simulink model "q1_b"  (R2026a)
settings: Solver=VariableStepAuto
model workspace (MAT data in the model file):
  K = Simulink.Parameter
  K.Complexity = 'real'
  K.Dimensions = [0 0]
  K.DataType = 'auto'
  K1 = Simulink.Parameter
  K1.Value = 4
  K1.Complexity = 'real'
  K1.Dimensions = [1 1]
  K1.DataType = 'auto'
  K1_2 = Simulink.Parameter
  K1_2.Value = 2
  K1_2.Complexity = 'real'
  K1_2.Dimensions = [1 1]
  K1_2.DataType = 'auto'
  K1_3 = Simulink.Parameter
  K1_3.Value = 5
  K1_3.Complexity = 'real'
  K1_3.Dimensions = [1 1]
  K1_3.DataType = 'auto'
  K2 = Simulink.Parameter
  K2.Value = 2
  K2.Complexity = 'real'
  K2.Dimensions = [1 1]
  K2.DataType = 'auto'
  K2_2 = Simulink.Parameter
  K2_2.Value = 4
  K2_2.Complexity = 'real'
  K2_2.Dimensions = [1 1]
  K2_2.DataType = 'auto'
  K2_3 = Simulink.Parameter
  K2_3.Value = 10
  K2_3.Complexity = 'real'
  K2_3.Dimensions = [1 1]
  K2_3.DataType = 'auto'
  a = Simulink.Parameter
  a.Value = 2
  a.Complexity = 'real'
  a.Dimensions = [1 1]
  a.DataType = 'auto'
settings Model: Creator=LAB_PC  LastModifiedBy=LAB_PC

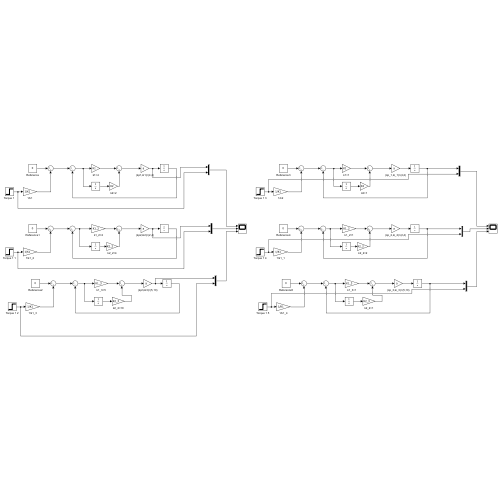
[thumbnail: Simulink's stored preview of the top-level diagram]
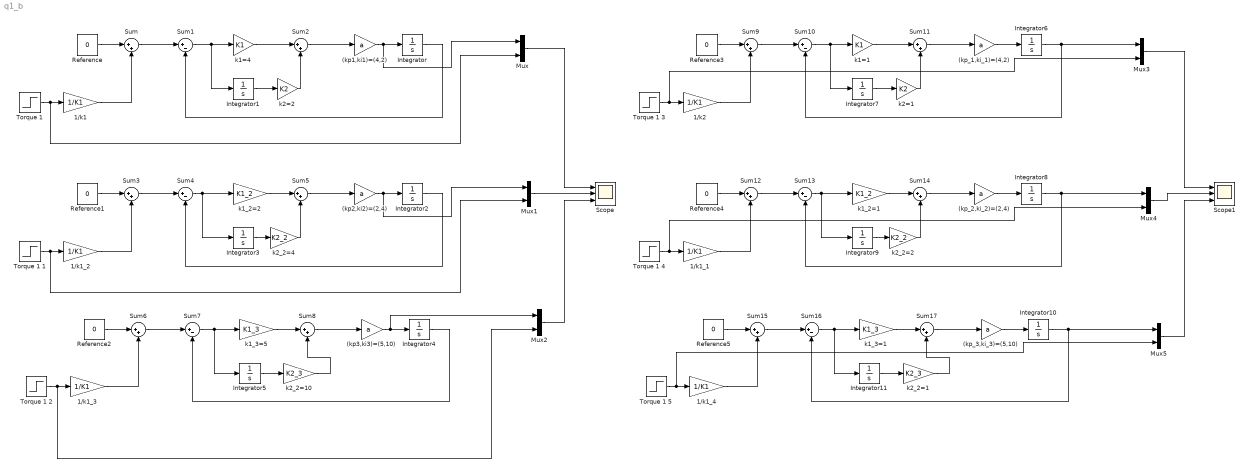
== system q1_b ==
  (kp1,ki1)=(4,2) : Gain  Gain=a
  (kp2,ki2)=(2,4) : Gain  Gain=a
  (kp3,ki3)=(5,10) : Gain  Gain=a
  (kp_1,ki_1)=(4,2) : Gain  Gain=a
  (kp_2,ki_2)=(2,4) : Gain  Gain=a
  (kp_3,ki_3)=(5,10) : Gain  Gain=a
  1/k1 : Gain  Gain=1/K1
  1/k1_{1..4} (4 alike) : Gain  Gain=1/K1
  1/k2 : Gain  Gain=1/K1
  Integrator{,1..11} (12 alike) : Integrator
  Mux{,1..5} (6 alike) : Mux  Inputs=2
  Reference{,1..5} (6 alike) : Constant  Value=0
  Scope : Scope  NumInputPorts=3
      settings: TimeAxisLabels=None  ActiveDisplayYMinimum=-3.7287146935324462  ActiveDisplayYMaximum=4.3917788582215262  DataLoggingVariableName=ScopeData2
  Scope1 : Scope  NumInputPorts=3
      settings: TimeAxisLabels=None  ActiveDisplayYMinimum=-3.7287146935324462  ActiveDisplayYMaximum=4.3917788582215262
  Sum{,2..3,5..6,8..9,11..12,14..15,17} (12 alike) : Sum  Inputs=|++
  Sum{1,4,7,10,13,16} (6 alike) : Sum  Inputs=|+-
  Torque 1 {,1..5} (6 alike) : Step  SampleTime=0
  k1=1 : Gain  Gain=K1
  k1=4 : Gain  Gain=K1
  k1_2=1 : Gain  Gain=K1_2
  k1_2=2 : Gain  Gain=K1_2
  k1_3=1 : Gain  Gain=K1_3
  k1_3=5 : Gain  Gain=K1_3
  k2=1 : Gain  Gain=K2
  k2=2 : Gain  Gain=K2
  k2_2=1 : Gain  Gain=K2_3
  k2_2=10 : Gain  Gain=K2_3
  k2_2=2 : Gain  Gain=K2_2
  k2_2=4 : Gain  Gain=K2_2
  wires:
  Integrator/1 -> Sum1/2
  Reference/1 -> Sum/1
  1/k1/1 -> Sum/2
  (kp1,ki1)=(4,2)/1 -> Mux/1, Integrator/1
  "Torque 1 "/1 -> Mux/2, 1/k1/1
  Mux/1 -> Scope/1
  Sum1/1 -> Integrator1/1, k1=4/1
  Sum/1 -> Sum1/1
  Integrator1/1 -> k2=2/1
  k2=2/1 -> Sum2/2
  k1=4/1 -> Sum2/1
  Sum2/1 -> (kp1,ki1)=(4,2)/1
  Integrator3/1 -> k2_2=4/1
  Sum3/1 -> Sum4/1
  Torque 1 1/1 -> Mux1/2, 1/k1_2/1
  k1_2=2/1 -> Sum5/1
  Sum5/1 -> (kp2,ki2)=(2,4)/1
  Integrator2/1 -> Sum4/2
  Reference1/1 -> Sum3/1
  Sum4/1 -> Integrator3/1, k1_2=2/1
  1/k1_2/1 -> Sum3/2
  k2_2=4/1 -> Sum5/2
  (kp2,ki2)=(2,4)/1 -> Mux1/1, Integrator2/1
  Sum6/1 -> Sum7/1
  (kp3,ki3)=(5,10)/1 -> Mux2/1, Integrator4/1
  k2_2=10/1 -> Sum8/2
  Sum7/1 -> Integrator5/1, k1_3=5/1
  1/k1_3/1 -> Sum6/2
  Integrator4/1 -> Sum7/2
  Reference2/1 -> Sum6/1
  Torque 1 2/1 -> Mux2/2, 1/k1_3/1
  Integrator5/1 -> k2_2=10/1
  k1_3=5/1 -> Sum8/1
  Sum8/1 -> (kp3,ki3)=(5,10)/1
  Mux1/1 -> Scope/2
  Mux2/1 -> Scope/3
  Mux4/1 -> Scope1/2
  Integrator6/1 -> Sum10/2, Mux3/1
  Sum14/1 -> (kp_2,ki_2)=(2,4)/1
  Integrator11/1 -> k2_2=1/1
  Sum11/1 -> (kp_1,ki_1)=(4,2)/1
  Torque 1 5/1 -> Mux5/2, 1/k1_4/1
  Mux5/1 -> Scope1/3
  (kp_3,ki_3)=(5,10)/1 -> Integrator10/1
  (kp_2,ki_2)=(2,4)/1 -> Integrator8/1
  Sum15/1 -> Sum16/1
  Sum12/1 -> Sum13/1
  Integrator7/1 -> k2=1/1
  Integrator8/1 -> Sum13/2, Mux4/1
  (kp_1,ki_1)=(4,2)/1 -> Integrator6/1
  Sum13/1 -> Integrator9/1, k1_2=1/1
  1/k2/1 -> Sum9/2
  k2_2=1/1 -> Sum17/2
  Reference5/1 -> Sum15/1
  Torque 1 4/1 -> Mux4/2, 1/k1_1/1
  Integrator10/1 -> Mux5/1, Sum16/2
  k1=1/1 -> Sum11/1
  Integrator9/1 -> k2_2=2/1
  k1_2=1/1 -> Sum14/1
  Sum16/1 -> Integrator11/1, k1_3=1/1
  Reference3/1 -> Sum9/1
  Sum17/1 -> (kp_3,ki_3)=(5,10)/1
  k1_3=1/1 -> Sum17/1
  Sum9/1 -> Sum10/1
  Torque 1 3/1 -> Mux3/2, 1/k2/1
  1/k1_1/1 -> Sum12/2
  Reference4/1 -> Sum12/1
  k2=1/1 -> Sum11/2
  1/k1_4/1 -> Sum15/2
  Sum10/1 -> Integrator7/1, k1=1/1
  Mux3/1 -> Scope1/1
  k2_2=2/1 -> Sum14/2
